simulink model "AMB_L_9_calibration_simulation"  (R2021a)
settings: Solver=ode4  StartTime=0.0  StopTime=tcal  FixedStep=dtsim  RelTol=1e-3
values from neighbouring files (symbols this model uses):
  adaptivegain = diag(10.^[8.4 6.2 2.1 0.8])    [AMB_L_1_vRTHS.m]    (also in AMB_L_2_calibration.m = gain2; AMB_L_5_optimization.m = diag(10.^op_location'); AMB_L_6_R2function.m = diag(10.^x); AMB_L_7_J2andInputs.m = diag(10.^x))
  Derivadas = [u;dudt;dudt2;dudt3]    [AMB_L_1_vRTHS.m]
  drefcal = 0.04    [AMB_L_2_calibration.m]
  dtsim = 1/fs    (= 0.000244140625)    [AMB_L_1_vRTHS.m]
  escala = 50/100    (= 0.5)    [AMB_L_1_vRTHS.m]    (also in AMB_L_2_calibration.m = 0.4)
  max_amb = [amb0max,amb1max,amb2max,amb3max]    [AMB_L_1_vRTHS.m]
  min_amb = [amb0min,amb1min,amb2min,amb3min]    [AMB_L_1_vRTHS.m]
  rms_noise_desp = 6.25e-14    [AMB_L_1_vRTHS.m]
  sat_limit_lower = -3.8    [AMB_L_1_vRTHS.m]
  sat_limit_upper = +3.8    (= 3.8)    [AMB_L_1_vRTHS.m]
  wnrefcal = 3.5*2*pi    (= 21.9911485751)    [AMB_L_2_calibration.m]
undefined symbols (not defined in the file or in its folder): dencal, denfilter, numcal, numfilter
libraries: simulink x1
settings Model: SimulationMode=accelerator  Creator=cristobal  LastModifiedBy=MSI
settings SolverCC: AlgebraicLoopSolver=TrustRegion
settings DataIOCC: ReturnWorkspaceOutputs=off
settings DebuggingCC: SFMachineParentedDataDiag=warning  ArithmeticOperatorsInVariantConditions=warning
settings SFSimCC: SimUseLocalCustomCode=off  CustomCodeUndefinedFunction=UseInterfaceOnly
settings RTWCC: RTWUseLocalCustomCode=off
settings CodeAppCC: StateflowObjectComments=on

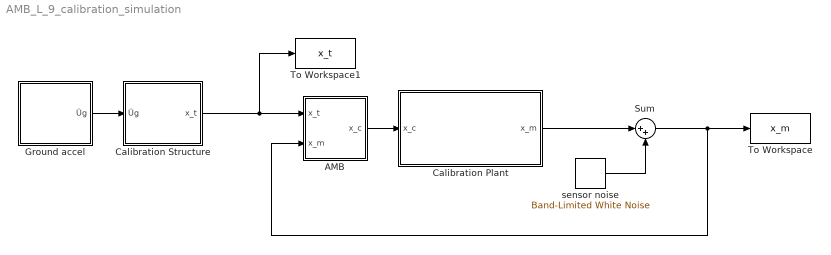
== system AMB_L_9_calibration_simulation ==
  AMB : Subsystem
  Calibration Plant : Subsystem
  Calibration Structure : Subsystem
  Ground accel : Subsystem
  Sum : Sum  Inputs=|++
  To Workspace : ToWorkspace  VariableName=x_m  SaveFormat=Timeseries  SampleTime=-1
  To Workspace1 : ToWorkspace  VariableName=x_t  SaveFormat=Timeseries  SampleTime=-1
  sensor noise : simulink/Sources/Band-Limited White Noise  Cov=[rms_noise_desp]  Ts=dtsim  seed=ceil(rand(1)*10000)
  wires:
  AMB/1(x_c) -> Calibration Plant/1(x_c)
  Calibration Plant/1(x_m) -> Sum/1
  Sum/1 -> To Workspace/1, AMB/2(x_m)
  Calibration Structure/1(x_t) -> AMB/1(x_t), To Workspace1/1
  Ground accel/1(Üg) -> Calibration Structure/1(Üg)
  sensor noise/1 -> Sum/2

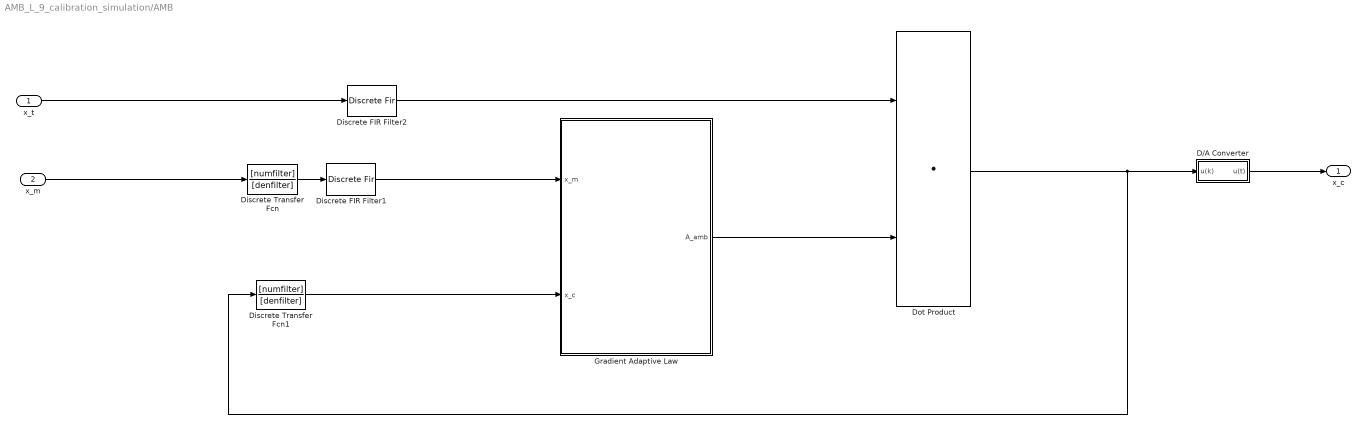
== system AMB_L_9_calibration_simulation/AMB ==
  x_t : Inport
  x_m : Inport  Port=2
  D/A Converter : Subsystem
  Discrete Transfer Fcn : DiscreteTransferFcn  Numerator=[numfilter]  Denominator=[denfilter]
  Discrete Transfer Fcn1 : DiscreteTransferFcn  Numerator=[numfilter]  Denominator=[denfilter]
  Discrete FIR Filter1 : DiscreteFir  Coefficients=Derivadas
  Discrete FIR Filter2 : DiscreteFir  Coefficients=Derivadas
  Dot Product : DotProduct  InputSameDT=on  OutDataTypeStr=Inherit: Inherit via internal rule
  Gradient Adaptive Law : Subsystem
  x_c : Outport  VectorParamsAs1DForOutWhenUnconnected=off
  wires:
  Gradient Adaptive Law/1(A_amb) -> Dot Product/2
  Discrete FIR Filter1/1 -> Gradient Adaptive Law/1(x_m)
  Discrete Transfer Fcn1/1 -> Gradient Adaptive Law/2(x_c)
  D/A Converter/1(u(t)) -> x_c/1
  x_m/1 -> Discrete Transfer Fcn/1
  Discrete Transfer Fcn/1 -> Discrete FIR Filter1/1
  x_t/1 -> Discrete FIR Filter2/1
  Dot Product/1 -> D/A Converter/1(u(k)), Discrete Transfer Fcn1/1
  Discrete FIR Filter2/1 -> Dot Product/1

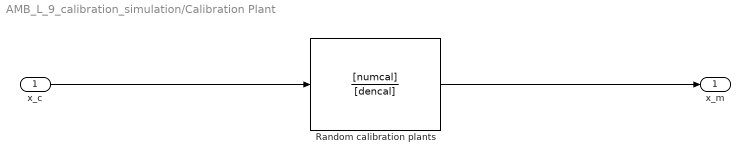
== system AMB_L_9_calibration_simulation/Calibration Plant ==
  x_c : Inport
  Random calibration plants : TransferFcn  Numerator=[numcal]  Denominator=[dencal]
  x_m : Outport  VectorParamsAs1DForOutWhenUnconnected=off
  wires:
  x_c/1 -> Random calibration plants/1
  Random calibration plants/1 -> x_m/1

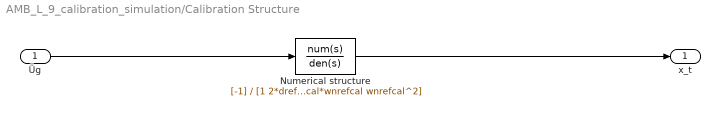
== system AMB_L_9_calibration_simulation/Calibration Structure ==
  Üg : Inport
  Numerical structure : TransferFcn  Numerator=[-1]  Denominator=[1 2*drefcal*wnrefcal wnrefcal^2]
  x_t : Outport  VectorParamsAs1DForOutWhenUnconnected=off
  wires:
  Üg/1 -> Numerical structure/1
  Numerical structure/1 -> x_t/1

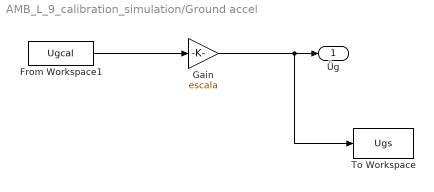
== system AMB_L_9_calibration_simulation/Ground accel ==
  From Workspace1 : FromWorkspace  VariableName=Ugcal  OutputAfterFinalValue=Setting to zero
  Gain : Gain  Gain=escala
  To Workspace : ToWorkspace  VariableName=Ugs  SaveFormat=Timeseries  SampleTime=-1
  Üg : Outport  VectorParamsAs1DForOutWhenUnconnected=off
  wires:
  From Workspace1/1 -> Gain/1
  Gain/1 -> To Workspace/1, Üg/1

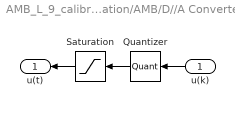
== system AMB_L_9_calibration_simulation/AMB/D//A Converter ==
  u(k) : Inport
  Quantizer : Quantizer  QuantizationInterval=quantize_int
  Saturation : Saturate  UpperLimit=sat_limit_upper  LowerLimit=sat_limit_lower
  u(t) : Outport  VectorParamsAs1DForOutWhenUnconnected=off
  wires:
  Saturation/1 -> u(t)/1
  Quantizer/1 -> Saturation/1
  u(k)/1 -> Quantizer/1

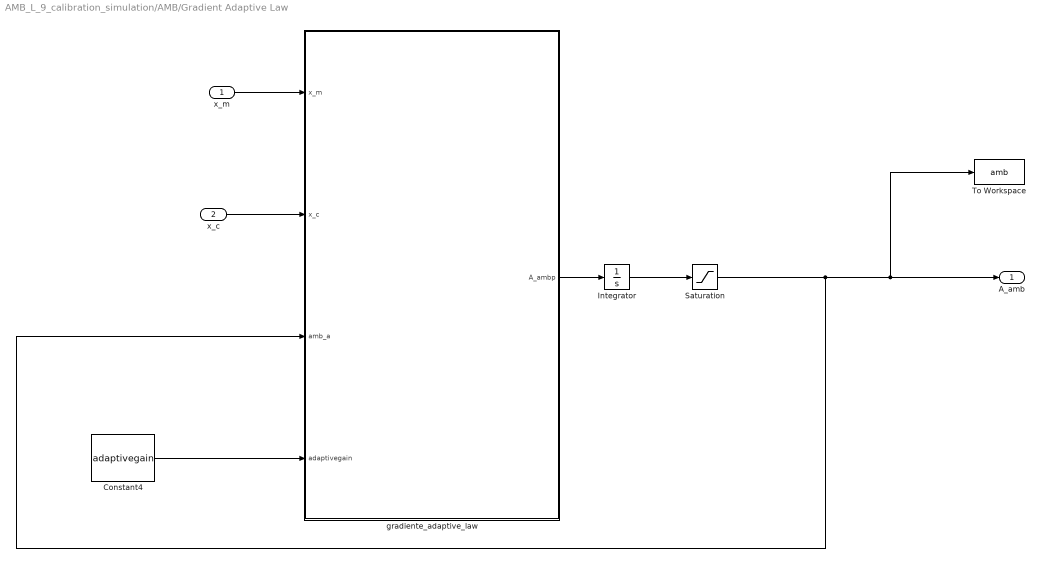
== system AMB_L_9_calibration_simulation/AMB/Gradient Adaptive Law ==
  x_m : Inport
  x_c : Inport  Port=2
  Constant4 : Constant  Value=adaptivegain
  Integrator : Integrator  InitialCondition=A_amb_i'
  Saturation : Saturate  UpperLimit=[max_amb]  LowerLimit=min_amb
  To Workspace : ToWorkspace  VariableName=amb  SaveFormat=Timeseries  SampleTime=-1
  gradiente_adaptive_law : MATLAB Function  TreatAsAtomicUnit=on
  A_amb : Outport  VectorParamsAs1DForOutWhenUnconnected=off
  wires:
  Saturation/1 -> gradiente_adaptive_law/3(amb_a), To Workspace/1, A_amb/1
  Integrator/1 -> Saturation/1
  x_c/1 -> gradiente_adaptive_law/2(x_c)
  Constant4/1 -> gradiente_adaptive_law/4(adaptivegain)
  gradiente_adaptive_law/1(A_ambp) -> Integrator/1
  x_m/1 -> gradiente_adaptive_law/1(x_m)

== matlab function AMB_L_9_calibration_simulation/AMB/Gradient Adaptive Law/gradiente_adaptive_law ==
  data: x_m input; x_c input; amb_a input; A_ambp output; adaptivegain input
function A_ambp   = fcn(x_m,x_c,amb_a,adaptivegain)
error=(x_c-amb_a'*x_m)/(1+(x_m'*x_m));
A_ambp=adaptivegain*error*x_m;
